simulink model "PROBLEM1"  (R2020b)
settings: Solver=VariableStepAuto  StartTime=0.0  StopTime=200  RelTol=1e-3
settings Model: Creator=Lenovo  LastModifiedBy=Lenovo

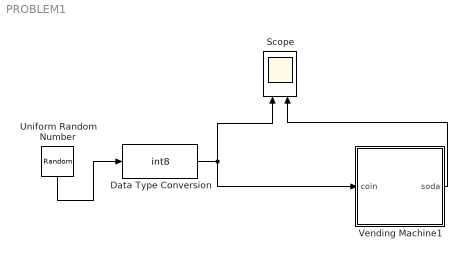
== system PROBLEM1 ==
  Data Type Conversion : DataTypeConversion  OutDataTypeStr=int8  RndMeth=Nearest  SaturateOnIntegerOverflow=on
  Scope : Scope  NumInputPorts=2
  Uniform Random Number : UniformRandomNumber  Minimum=0  Maximum=2  Seed=337  SampleTime=10
  Vending Machine1 : Stateflow chart  TreatAsAtomicUnit=on
  wires:
  Data Type Conversion/1 -> Vending Machine1/1(coin), Scope/1
  Vending Machine1/1(soda) -> Scope/2
  Uniform Random Number/1 -> Data Type Conversion/1

== stateflow chart PROBLEM1/Vending Machine1 ==
  state got_0
  state got_nickel
  state got_dime
  (default) -> got_0
  got_0 -> got_nickel [order 1] : [coin==1]{soda=0}
  got_nickel -> got_0 [order 2] : [coin==2]{soda=1}
  got_dime -> got_0 [order 1] : [coin==1]{soda=1}
  got_0 -> got_dime [order 2] : [coin==2]{soda=0}
  got_dime -> got_nickel [order 2] : [coin==2]{soda=1}
  got_nickel -> got_dime [order 1] : [coin==1]{soda=0}
  data: soda output; coin input
